simulink library "Valve_Thermostatic"  (Simulink 8.2)
settings: Solver=ode45  StartTime=0.0  StopTime=10.0  RelTol=1e-3
libraries: carnot x1
settings Model: Creator=lena.frank  LastModifiedBy=drhf

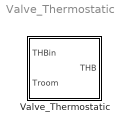
== system Valve_Thermostatic ==
  Valve_Thermostatic : Subsystem  mask(thermostatic valve){Tset=20, prange=3, op=0.5, bl=0.1, ts=30, dia=0.02, vpos=[0 0.1 1], vqua=[1e6 1e6 1]}
      mask prompts: Tset "set temperature [degree centigrade]"; prange "proportional Range [K]"; op "operating point [0..1] (valve position at set temperature)"; bl "play hysterersis in K"; ts "first-order hold ts [s]"; dia "diameter [m]"; vpos "Valve position vector [0..1]"; vqua "Vector with quadratic pressure drop in massflow in Pa*s²/kg²"
      mask help:
      | Thermostatic valve for a radiator.
      | set temperature and slope
      | valve position = -slope * (T(sensor) - Toffset)
      mask Help: web(fullfile(path_carnot('help'),'Valve_Thermostatic.html'),'-helpbrowser')
      mask Display:
      | plot(-20,-10,130,110,[20,80,80,20,20],[60,30,60,30,60],[50,50],[45,70],[60,40],[96,96],[50,50],[75,96])
      | port_label('input',1,'THB')
      | port_label('input',2,'Troom')
      | port_label('output',1,'THB')

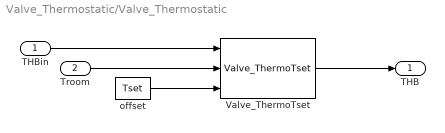
== system Valve_Thermostatic/Valve_Thermostatic ==
  THBin : Inport
  Troom : Inport  Port=2
  Valve_ThermoTset : carnot/Hydraulics/Valve_ThermoTset  p=prange  op=op  bl=bl  ts=ts  dia=dia  vpos=vpos  vqua=vqua
  offset : Constant  Value=Tset
  THB : Outport
  wires:
  Valve_ThermoTset/1 -> THB/1
  THBin/1 -> Valve_ThermoTset/1
  Troom/1 -> Valve_ThermoTset/2
  offset/1 -> Valve_ThermoTset/3
